simulink model "simulation_model_PD_tuning"  (R2021b)
settings: Solver=VariableStepAuto  StartTime=0.0  StopTime=10  MaxStep=1e-4  RelTol=1e-5
settings Model: Creator=Mohamad Chehadeh  LastModifiedBy=Admin
settings SolverCC: AlgebraicLoopSolver=TrustRegion
settings DebuggingCC: SFMachineParentedDataDiag=warning

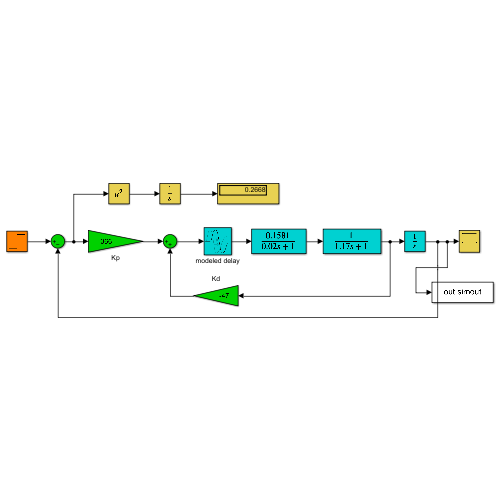
[thumbnail: Simulink's stored preview of the top-level diagram]
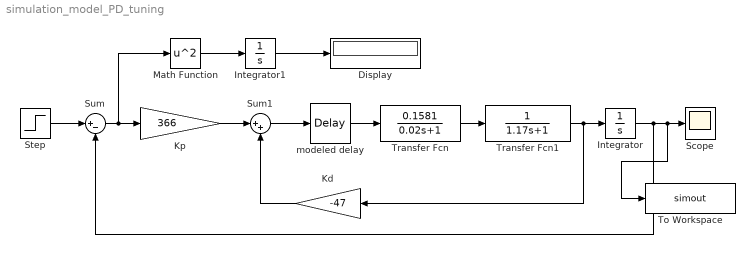
== system simulation_model_PD_tuning ==
  Display : Display
  Integrator : Integrator
  Integrator1 : Integrator
  Kd : Gain  Gain=-47
  Kp : Gain  Gain=366
  Math Function : Math  Operator=square  SaturateOnIntegerOverflow=on
  Scope : Scope
  Step : Step  SampleTime=0
  Sum : Sum  Inputs=|+-
  Sum1 : Sum  Inputs=|++
  To Workspace : ToWorkspace  VariableName=simout  SaveFormat=Timeseries  SampleTime=-1
  Transfer Fcn : TransferFcn  Numerator=[0.1581]  Denominator=[0.02 1]
  Transfer Fcn1 : TransferFcn  Denominator=[1.17 1]
  modeled delay : TransportDelay  DelayTime=0.060739
  wires:
  Math Function/1 -> Integrator1/1
  Integrator1/1 -> Display/1
  Transfer Fcn/1 -> Transfer Fcn1/1
  Kd/1 -> Sum1/2
  Transfer Fcn1/1 -> Integrator/1, Kd/1
  Integrator/1 -> To Workspace/1, Scope/1, Sum/2
  Kp/1 -> Sum1/1
  Sum/1 -> Kp/1, Math Function/1
  Step/1 -> Sum/1
  Sum1/1 -> modeled delay/1
  modeled delay/1 -> Transfer Fcn/1
